simulink model "P2D_JustPlantStep_NoNoise_NoVarInput_sine"  (R2022a)
settings: Solver=VariableStepAuto  StartTime=0.0  StopTime=10  RelTol=1e-3
settings Model: Creator=tyevans  LastModifiedBy=tyevans

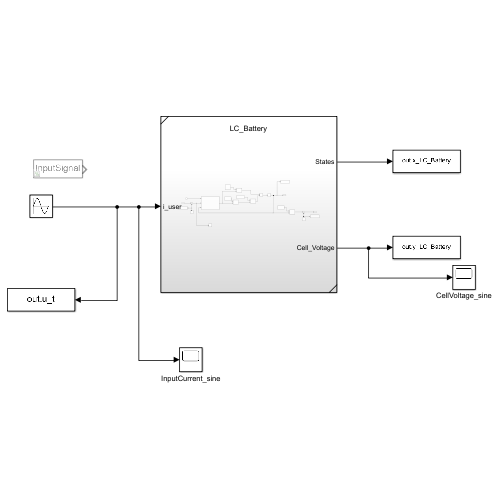
[thumbnail: Simulink's stored preview of the top-level diagram]
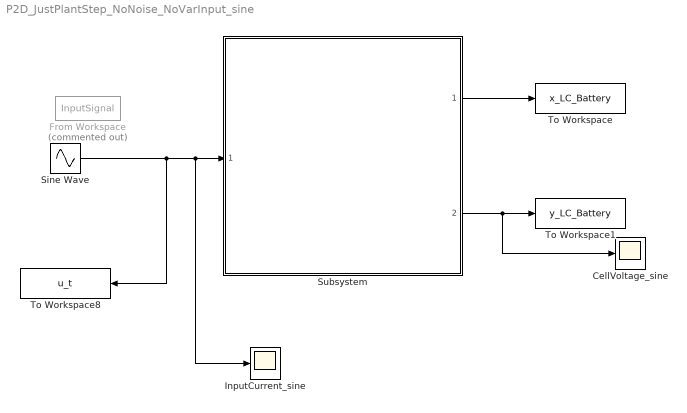
== system P2D_JustPlantStep_NoNoise_NoVarInput_sine ==
  CellVoltage_sine : Scope
  From Workspace : FromWorkspace  Commented=on  VariableName=InputSignal  OutputAfterFinalValue=Setting to zero
  InputCurrent_sine : Scope
  Sine Wave : Sin  Frequency=2*pi  SampleTime=0
  Subsystem : Subsystem  ReferencedSubsystem=LC_Battery
  To Workspace : ToWorkspace  VariableName=x_LC_Battery  SaveFormat=Structure With Time  SampleTime=-1
  To Workspace1 : ToWorkspace  VariableName=y_LC_Battery  SaveFormat=Structure With Time  SampleTime=-1
  To Workspace8 : ToWorkspace  VariableName=u_t  SaveFormat=Structure With Time  SampleTime=-1
  wires:
  Subsystem/1 -> To Workspace/1
  Subsystem/2 -> To Workspace1/1, CellVoltage_sine/1
  Sine Wave/1 -> To Workspace8/1, InputCurrent_sine/1, Subsystem/1
